simulink model "ex_8_3"  (Simulink 10.1)
settings: Solver=FixedStepAuto  StartTime=0.0  StopTime=10  FixedStep=0.01  RelTol=1e-3
settings Model: Creator=Paulo Padrao  LastModifiedBy=Paulo Padrao
settings DataIOCC: SaveFormat=Dataset
settings OptimizationCC: LifeSpan=auto
settings DebuggingCC: UnderspecifiedInitializationDetection=Simplified  MergeDetectMultiDrivingBlocksExec=error  SFUnexpectedBacktrackingDiag=error  SFNoUnconditionalDefaultTransitionDiag=error  SFExecutionAtInitializationDiag=warning
settings HardwareCC: ProdBitPerPointer=64  ProdBitPerSizeT=64  ProdBitPerPtrDiffT=64  ProdLargestAtomicFloat=Float  ProdIntDivRoundTo=Zero  ProdEndianess=LittleEndian  ProdWordSize=64  ProdHWDeviceType=Intel->x86-64 (Windows64)
settings ModelReferenceCC: PropagateSignalLabelsOutOfModel=on
settings CodeAppCC: StateflowObjectComments=off
settings GRTTargetCC: TargetLangStandard=C99 (ISO)  CombineOutputUpdateFcns=on  GRTInterface=off
settings ConfigComp: CovMetricSettings=dwe  CovHtmlReporting=off  CovSaveCumulativeToWorkspaceVar=off  CovSaveSingleToWorkspaceVar=off  CovExternalEMLEnable=on

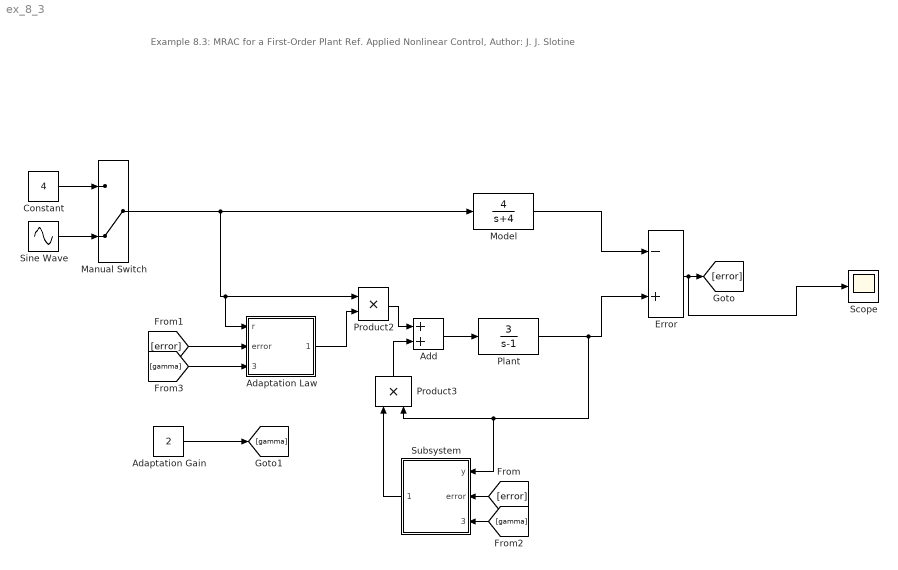
== system ex_8_3 ==
  note: Example 8.3: MRAC for a First-Order Plant
      |
      | Ref. Applied Nonlinear Control, Author: J. J. Slotine
  "Adaptation Gain " : Constant  Value=2
  Adaptation Law : Subsystem
  Add : Sum
  Constant : Constant  Value=4
  Error : Sum  Inputs=-+
  Manual Switch : ManualSwitch  CurrentSetting=0
  Model : TransferFcn  Numerator=[4]  Denominator=[1 4]
  Plant : TransferFcn  Numerator=[3]  Denominator=[1 -1]
  Product2 : Product
  Product3 : Product
  Scope : Scope
  Sine Wave : Sin  Amplitude=4  Frequency=3  SampleTime=0
  Subsystem : Subsystem
  wires:
  Model/1 -> Error/1
  Plant/1 -> Subsystem/1(y), Product3/2, Error/2
  Constant/1 -> Manual Switch/1
  Sine Wave/1 -> Manual Switch/2
  Manual Switch/1 -> Model/1, Adaptation Law/1(r), Product2/1
  Add/1 -> Plant/1
  Error/1 -> Scope/1, [error]
  "Adaptation Gain "/1 -> [gamma]
  Product2/1 -> Add/1
  Product3/1 -> Add/2
  Adaptation Law/1(ar_hat) -> Product2/2
  [error] -> Adaptation Law/2(error)
  [gamma] -> Adaptation Law/3(gamma)
  Subsystem/1(ay_hat) -> Product3/1
  [error] -> Subsystem/2(error)
  [gamma] -> Subsystem/3(gamma)

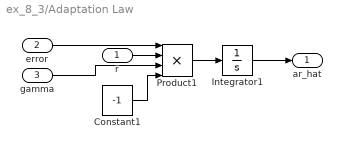
== system ex_8_3/Adaptation Law ==
  r : Inport
  error : Inport  Port=2
  gamma : Inport  Port=3
  Constant1 : Constant  Value=-1
  Integrator1 : Integrator
  Product1 : Product  Inputs=4
  ar_hat : Outport  VectorParamsAs1DForOutWhenUnconnected=off
  wires:
  Integrator1/1 -> ar_hat/1
  error/1 -> Product1/1
  r/1 -> Product1/2
  gamma/1 -> Product1/3
  Product1/1 -> Integrator1/1
  Constant1/1 -> Product1/4

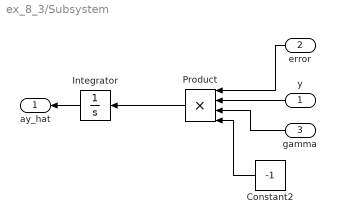
== system ex_8_3/Subsystem ==
  y : Inport
  error : Inport  Port=2
  gamma : Inport  Port=3
  Constant2 : Constant  Value=-1
  Integrator : Integrator
  Product : Product  Inputs=4
  ay_hat : Outport  VectorParamsAs1DForOutWhenUnconnected=off
  wires:
  error/1 -> Product/1
  y/1 -> Product/2
  Constant2/1 -> Product/4
  Integrator/1 -> ay_hat/1
  gamma/1 -> Product/3
  Product/1 -> Integrator/1
